simulink model "PIDcontrol"  (R2023b)
settings: Solver=VariableStepAuto  StartTime=0.0  StopTime=4  RelTol=1e-3
undefined symbols (not defined in the file or in its folder): my_gravity_torque, my_mass_matrix, my_velocity_product
settings Model: Creator=孙伟杰  LastModifiedBy=孙伟杰

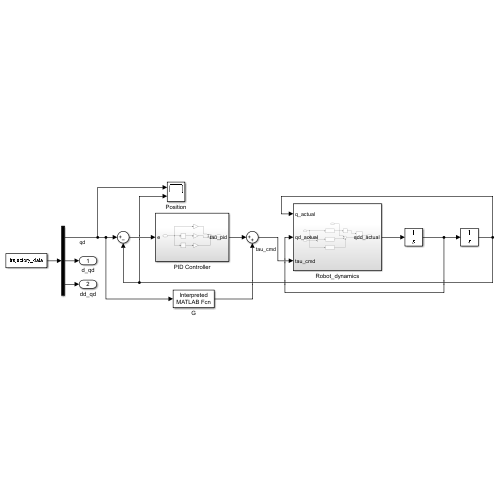
[thumbnail: Simulink's stored preview of the top-level diagram]
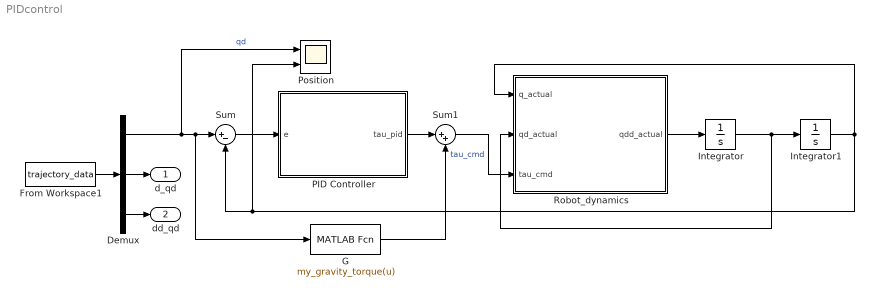
== system PIDcontrol ==
  Demux : Demux  Outputs=[6 6 6]
  From Workspace1 : FromWorkspace  VariableName=trajectory_data  SampleTime=-1
  G : MATLABFcn  MATLABFcn=my_gravity_torque(u)  OutputDimensions=6
  Integrator : Integrator
  Integrator1 : Integrator
  PID Controller : Subsystem
  Position : Scope  NumInputPorts=2
  Robot_dynamics : Subsystem
  Sum : Sum  Inputs=|+-
  Sum1 : Sum  Inputs=|++
  d_qd : Outport
  dd_qd : Outport  Port=2
  wires:
  Sum/1 -> PID Controller/1(e)
  PID Controller/1(tau_pid) -> Sum1/1
  G/1 -> Sum1/2
  Sum1/1 -> Robot_dynamics/3(tau_cmd)  "tau_cmd"
  Robot_dynamics/1(qdd_actual) -> Integrator/1
  Integrator/1 -> Robot_dynamics/2(qd_actual), Integrator1/1
  Integrator1/1 -> Position/2, Sum/2, Robot_dynamics/1(q_actual)
  From Workspace1/1 -> Demux/1
  Demux/1 -> G/1, Sum/1, Position/1  "qd"
  Demux/2 -> d_qd/1
  Demux/3 -> dd_qd/1

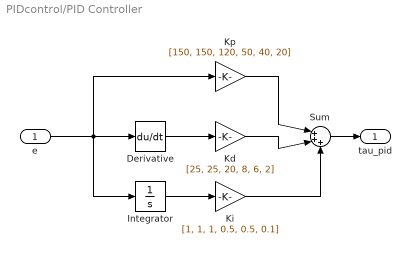
== system PIDcontrol/PID Controller ==
  e : Inport
  Derivative : Derivative
  Integrator : Integrator
  Kd : Gain  Gain=[25, 25, 20, 8, 6, 2]
  Ki : Gain  Gain=[1, 1, 1, 0.5, 0.5, 0.1]
  Kp : Gain  Gain=[150, 150, 120, 50, 40, 20]
  Sum : Sum  Inputs=|+++
  tau_pid : Outport
  wires:
  Derivative/1 -> Kd/1
  Integrator/1 -> Ki/1
  Kp/1 -> Sum/1
  Kd/1 -> Sum/2
  Ki/1 -> Sum/3
  Sum/1 -> tau_pid/1
  e/1 -> Integrator/1, Derivative/1, Kp/1

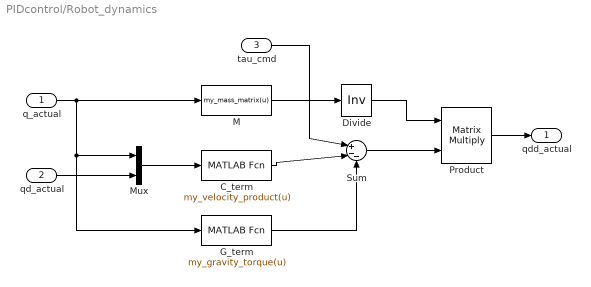
== system PIDcontrol/Robot_dynamics ==
  q_actual : Inport
  qd_actual : Inport  Port=2
  tau_cmd : Inport  Port=3
  C_term : MATLABFcn  MATLABFcn=my_velocity_product(u)  OutputDimensions=6
  Divide : Product  Inputs=/  Multiplication=Matrix(*)
  G_term : MATLABFcn  MATLABFcn=my_gravity_torque(u)  OutputDimensions=6
  M : MATLABFcn  MATLABFcn=my_mass_matrix(u)  OutputDimensions=[6 6]  Output1D=off
  Mux : Mux  Inputs=2
  Product : Product  Multiplication=Matrix(*)
  Sum : Sum  Inputs=|+--
  qdd_actual : Outport
  wires:
  q_actual/1 -> G_term/1, Mux/1, M/1
  Mux/1 -> C_term/1
  qd_actual/1 -> Mux/2
  tau_cmd/1 -> Sum/1
  C_term/1 -> Sum/2
  G_term/1 -> Sum/3
  M/1 -> Divide/1
  Sum/1 -> Product/2
  Divide/1 -> Product/1
  Product/1 -> qdd_actual/1
